simulink model "CAM_Example"  (R2021a)
settings: Solver=VariableStepAuto  StartTime=0.0  StopTime=10.0  RelTol=1e-3
libraries: c2xlib x29
settings Model: EnablePacing=on  Creator=User  LastModifiedBy=User

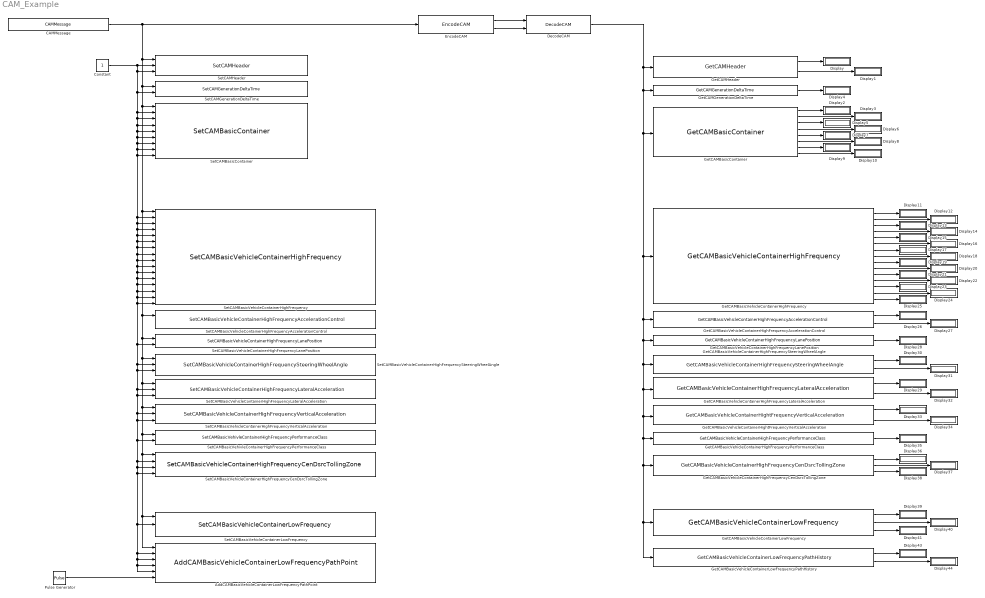
== system CAM_Example ==
  AddCAMBasicVehicleContainerLowFrequencyPathPoint : c2xlib/AddCAMBasicVehicleContainerLowFrequencyPathPoint  SimulateUsing=Code generation
      settings: SourceProductName=C2XLib
  CAMMessage : c2xlib/CAMMessage  StationID=0  HeighFrequencyContainerType=0  SimulateUsing=Code generation
      settings: SourceProductName=C2XLib
  Constant : Constant
  DecodeCAM : c2xlib/DecodeCAM  SimulateUsing=Code generation
      settings: SourceProductName=C2XLib
  Display{,1..41,43..44} (44 alike) : Display
  EncodeCAM : c2xlib/EncodeCAM  BufferSize=65535  SimulateUsing=Code generation
      settings: SourceProductName=C2XLib
  GetCAMBasicContainer : c2xlib/GetCAMBasicContainer  SimulateUsing=Code generation
      settings: SourceProductName=C2XLib
  GetCAMBasicVehicleContainerHighFrequency : c2xlib/GetCAMBasicVehicleContainerHighFrequency  SimulateUsing=Code generation
      settings: SourceProductName=C2XLib
  GetCAMBasicVehicleContainerHighFrequencyAccelerationControl : c2xlib/GetCAMBasicVehicleContainerHighFrequencyAccelerationControl  BufferSize=0  SimulateUsing=Code generation
      settings: SourceProductName=C2XLib
  GetCAMBasicVehicleContainerHighFrequencyCenDsrcTollingZone : c2xlib/GetCAMBasicVehicleContainerHighFrequencyCenDsrcTollingZone  SimulateUsing=Code generation
      settings: SourceProductName=C2XLib
  GetCAMBasicVehicleContainerHighFrequencyLanePosition : c2xlib/GetCAMBasicVehicleContainerHighFrequencyLanePosition  SimulateUsing=Code generation
      settings: SourceProductName=C2XLib
  GetCAMBasicVehicleContainerHighFrequencyLateralAcceleration : c2xlib/GetCAMBasicVehicleContainerHighFrequencyLateralAcceleration  SimulateUsing=Code generation
      settings: SourceProductName=C2XLib
  GetCAMBasicVehicleContainerHighFrequencyPerformanceClass : c2xlib/GetCAMBasicVehicleContainerHighFrequencyPerformanceClass  SimulateUsing=Code generation
      settings: SourceProductName=C2XLib
  GetCAMBasicVehicleContainerHighFrequencySteeringWheelAngle : c2xlib/GetCAMBasicVehicleContainerHighFrequencySteeringWheelAngle  SimulateUsing=Code generation
      settings: SourceProductName=C2XLib
  GetCAMBasicVehicleContainerHightFrequencyVerticalAcceleration : c2xlib/GetCAMBasicVehicleContainerHightFrequencyVerticalAcceleration  SimulateUsing=Code generation
      settings: SourceProductName=C2XLib
  GetCAMBasicVehicleContainerLowFrequency : c2xlib/GetCAMBasicVehicleContainerLowFrequency  ExteriorLightsSize=2  SimulateUsing=Code generation
      settings: SourceProductName=C2XLib
  GetCAMBasicVehicleContainerLowFrequencyPathHistory : c2xlib/GetCAMBasicVehicleContainerLowFrequencyPathHistory  PathHistorySize=1  SimulateUsing=Code generation
      settings: SourceProductName=C2XLib
  GetCAMGenerationDeltaTime : c2xlib/GetCAMGenerationDeltaTime  SimulateUsing=Code generation
      settings: SourceProductName=C2XLib
  GetCAMHeader : c2xlib/GetCAMHeader  SimulateUsing=Code generation
      settings: SourceProductName=C2XLib
  Pulse Generator : DiscretePulseGenerator  PulseType=Time based  Period=5  PulseWidth=50  PhaseDelay=1
  SetCAMBasicContainer : c2xlib/SetCAMBasicContainer  SimulateUsing=Code generation
      settings: SourceProductName=C2XLib
  SetCAMBasicVehicleContainerHighFrequency : c2xlib/SetCAMBasicVehicleContainerHighFrequency  SimulateUsing=Code generation
      settings: SourceProductName=C2XLib
  SetCAMBasicVehicleContainerHighFrequencyAccelerationControl : c2xlib/SetCAMBasicVehicleContainerHighFrequencyAccelerationControl  SimulateUsing=Code generation
      settings: SourceProductName=C2XLib
  SetCAMBasicVehicleContainerHighFrequencyCenDsrcTollingZone : c2xlib/SetCAMBasicVehicleContainerHighFrequencyCenDsrcTollingZone  SimulateUsing=Code generation
      settings: SourceProductName=C2XLib
  SetCAMBasicVehicleContainerHighFrequencyLanePosition : c2xlib/SetCAMBasicVehicleContainerHighFrequencyLanePosition  SimulateUsing=Code generation
      settings: SourceProductName=C2XLib
  SetCAMBasicVehicleContainerHighFrequencyLateralAcceleration : c2xlib/SetCAMBasicVehicleContainerHighFrequencyLateralAcceleration  SimulateUsing=Code generation
      settings: SourceProductName=C2XLib
  SetCAMBasicVehicleContainerHighFrequencySteeringWheelAngle : c2xlib/SetCAMBasicVehicleContainerHighFrequencySteeringWheelAngle  SimulateUsing=Code generation
      settings: SourceProductName=C2XLib
  SetCAMBasicVehicleContainerHighFrequencyVerticalAcceleration : c2xlib/SetCAMBasicVehicleContainerHighFrequencyVerticalAcceleration  SimulateUsing=Code generation
      settings: SourceProductName=C2XLib
  SetCAMBasicVehicleContainerLowFrequency : c2xlib/SetCAMBasicVehicleContainerLowFrequency  SimulateUsing=Code generation
      settings: SourceProductName=C2XLib
  SetCAMBasicVehivleContainerHighFrequencyPerformanceClass : c2xlib/SetCAMBasicVehivleContainerHighFrequencyPerformanceClass  SimulateUsing=Code generation
      settings: SourceProductName=C2XLib
  SetCAMGenerationDeltaTime : c2xlib/SetCAMGenerationDeltaTime  SimulateUsing=Code generation
      settings: SourceProductName=C2XLib
  SetCAMHeader : c2xlib/SetCAMHeader  SimulateUsing=Code generation
      settings: SourceProductName=C2XLib
  wires:
  EncodeCAM/2 -> DecodeCAM/2
  EncodeCAM/1 -> DecodeCAM/1
  CAMMessage/1 -> AddCAMBasicVehicleContainerLowFrequencyPathPoint/1, SetCAMBasicVehicleContainerLowFrequency/1, SetCAMBasicVehicleContainerHighFrequencyCenDsrcTollingZone/1, SetCAMBasicVehivleContainerHighFrequencyPerformanceClass/1, SetCAMBasicVehicleContainerHighFrequencyVerticalAcceleration/1, SetCAMBasicVehicleContainerHighFrequencyLateralAcceleration/1, SetCAMBasicVehicleContainerHighFrequencySteeringWheelAngle/1, SetCAMBasicVehicleContainerHighFrequencyLanePosition/1, SetCAMBasicVehicleContainerHighFrequencyAccelerationControl/1, SetCAMBasicVehicleContainerHighFrequency/1, SetCAMBasicContainer/1, SetCAMGenerationDeltaTime/1, SetCAMHeader/1, EncodeCAM/1
  DecodeCAM/1 -> GetCAMBasicVehicleContainerLowFrequencyPathHistory/1, GetCAMBasicVehicleContainerLowFrequency/1, GetCAMBasicVehicleContainerHighFrequencyCenDsrcTollingZone/1, GetCAMBasicVehicleContainerHighFrequencyPerformanceClass/1, GetCAMBasicVehicleContainerHightFrequencyVerticalAcceleration/1, GetCAMBasicVehicleContainerHighFrequencyLateralAcceleration/1, GetCAMBasicVehicleContainerHighFrequencySteeringWheelAngle/1, GetCAMBasicVehicleContainerHighFrequencyLanePosition/1, GetCAMBasicVehicleContainerHighFrequencyAccelerationControl/1, GetCAMBasicVehicleContainerHighFrequency/1, GetCAMBasicContainer/1, GetCAMGenerationDeltaTime/1, GetCAMHeader/1
  Constant/1 -> AddCAMBasicVehicleContainerLowFrequencyPathPoint/5, AddCAMBasicVehicleContainerLowFrequencyPathPoint/4, AddCAMBasicVehicleContainerLowFrequencyPathPoint/3, AddCAMBasicVehicleContainerLowFrequencyPathPoint/2, SetCAMBasicVehicleContainerLowFrequency/2, SetCAMBasicVehicleContainerHighFrequencyCenDsrcTollingZone/4, SetCAMBasicVehicleContainerHighFrequencyCenDsrcTollingZone/3, SetCAMBasicVehicleContainerHighFrequencyCenDsrcTollingZone/2, SetCAMBasicVehivleContainerHighFrequencyPerformanceClass/2, SetCAMBasicVehicleContainerHighFrequencyVerticalAcceleration/3, SetCAMBasicVehicleContainerHighFrequencyVerticalAcceleration/2, SetCAMBasicVehicleContainerHighFrequencyLateralAcceleration/3, SetCAMBasicVehicleContainerHighFrequencyLateralAcceleration/2, SetCAMBasicVehicleContainerHighFrequencySteeringWheelAngle/3, SetCAMBasicVehicleContainerHighFrequencySteeringWheelAngle/2, SetCAMBasicVehicleContainerHighFrequencyLanePosition/2, SetCAMBasicVehicleContainerHighFrequency/16, SetCAMBasicVehicleContainerHighFrequency/15, SetCAMBasicVehicleContainerHighFrequency/14, SetCAMBasicVehicleContainerHighFrequency/13, SetCAMBasicVehicleContainerHighFrequency/12, SetCAMBasicVehicleContainerHighFrequency/11, SetCAMBasicVehicleContainerHighFrequency/10, SetCAMBasicVehicleContainerHighFrequency/9, SetCAMBasicVehicleContainerHighFrequency/8, SetCAMBasicVehicleContainerHighFrequency/7, SetCAMBasicVehicleContainerHighFrequency/6, SetCAMBasicVehicleContainerHighFrequency/5, SetCAMBasicVehicleContainerHighFrequency/4, SetCAMBasicVehicleContainerHighFrequency/3, SetCAMBasicVehicleContainerHighFrequency/2, SetCAMBasicContainer/9, SetCAMBasicContainer/8, SetCAMBasicContainer/7, SetCAMBasicContainer/6, SetCAMBasicContainer/5, SetCAMBasicContainer/4, SetCAMBasicContainer/3, SetCAMBasicContainer/2, SetCAMGenerationDeltaTime/2, SetCAMHeader/3, SetCAMHeader/2
  GetCAMHeader/2 -> Display1/1
  GetCAMHeader/1 -> Display/1
  GetCAMBasicContainer/2 -> Display3/1
  GetCAMBasicContainer/1 -> Display2/1
  GetCAMGenerationDeltaTime/1 -> Display4/1
  GetCAMBasicContainer/3 -> Display5/1
  GetCAMBasicContainer/4 -> Display6/1
  GetCAMBasicContainer/5 -> Display7/1
  GetCAMBasicContainer/6 -> Display8/1
  GetCAMBasicContainer/7 -> Display9/1
  GetCAMBasicContainer/8 -> Display10/1
  GetCAMBasicVehicleContainerHighFrequency/1 -> Display11/1
  GetCAMBasicVehicleContainerHighFrequency/2 -> Display12/1
  GetCAMBasicVehicleContainerHighFrequency/3 -> Display13/1
  GetCAMBasicVehicleContainerHighFrequency/4 -> Display14/1
  GetCAMBasicVehicleContainerHighFrequency/5 -> Display15/1
  GetCAMBasicVehicleContainerHighFrequency/6 -> Display16/1
  GetCAMBasicVehicleContainerHighFrequency/11 -> Display21/1
  GetCAMBasicVehicleContainerHighFrequency/12 -> Display22/1
  GetCAMBasicVehicleContainerHighFrequency/7 -> Display17/1
  GetCAMBasicVehicleContainerHighFrequency/10 -> Display20/1
  GetCAMBasicVehicleContainerHighFrequency/8 -> Display18/1
  GetCAMBasicVehicleContainerHighFrequency/9 -> Display19/1
  GetCAMBasicVehicleContainerHighFrequency/13 -> Display23/1
  GetCAMBasicVehicleContainerHighFrequency/14 -> Display24/1
  GetCAMBasicVehicleContainerHighFrequency/15 -> Display25/1
  GetCAMBasicVehicleContainerHighFrequencyAccelerationControl/2 -> Display27/1
  GetCAMBasicVehicleContainerHighFrequencyAccelerationControl/1 -> Display26/1
  GetCAMBasicVehicleContainerHighFrequencyLanePosition/1 -> Display28/1
  GetCAMBasicVehicleContainerHighFrequencySteeringWheelAngle/1 -> Display30/1
  GetCAMBasicVehicleContainerHighFrequencySteeringWheelAngle/2 -> Display31/1
  GetCAMBasicVehicleContainerHighFrequencyLateralAcceleration/2 -> Display32/1
  GetCAMBasicVehicleContainerHighFrequencyLateralAcceleration/1 -> Display29/1
  GetCAMBasicVehicleContainerHightFrequencyVerticalAcceleration/2 -> Display34/1
  GetCAMBasicVehicleContainerHightFrequencyVerticalAcceleration/1 -> Display33/1
  GetCAMBasicVehicleContainerHighFrequencyPerformanceClass/1 -> Display35/1
  GetCAMBasicVehicleContainerHighFrequencyCenDsrcTollingZone/1 -> Display36/1
  GetCAMBasicVehicleContainerHighFrequencyCenDsrcTollingZone/2 -> Display37/1
  GetCAMBasicVehicleContainerHighFrequencyCenDsrcTollingZone/3 -> Display38/1
  GetCAMBasicVehicleContainerLowFrequency/1 -> Display39/1
  GetCAMBasicVehicleContainerLowFrequency/2 -> Display40/1
  GetCAMBasicVehicleContainerLowFrequency/3 -> Display41/1
  GetCAMBasicVehicleContainerLowFrequencyPathHistory/1 -> Display43/1
  GetCAMBasicVehicleContainerLowFrequencyPathHistory/2 -> Display44/1
  Pulse Generator/1 -> AddCAMBasicVehicleContainerLowFrequencyPathPoint/6
